simulink model "sf_tlbefore"  (Simulink 7.6)
settings: Solver=ode45  StartTime=0.0  StopTime=20  MaxStep=.01  RelTol=1e-3
settings Model: Creator=The MathWorks Inc.  CovMetricSettings=dcmtr  ExtModeAutoUpdateStatusClock=off
settings OptimizationCC: BooleanDataType=off  InlineInvariantSignals=on  InitFltsAndDblsToZero=on  EfficientMapNaN2IntZero=off
settings DebuggingCC: SaveWithParameterizedLinksMsg=none  SignalResolutionControl=TryResolveAllWithWarning  SolverPrmCheckMsg=none  MultiTaskDSMMsg=warning  MultiTaskCondExecSysMsg=none  StrictBusMsg=None
settings HardwareCC: TargetUnknown=on
settings SFSimCC: SimParseCustomCode=off
settings RTWCC: IncludeERTFirstTime=on
settings GRTTargetCC: TargetFcnLib=ansi_tfl_tmw.mat

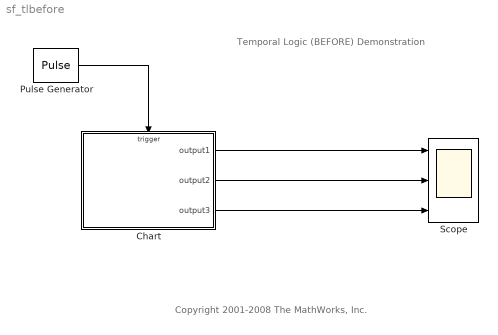
== system sf_tlbefore ==
  note: Temporal Logic (BEFORE) Demonstration
  note: Copyright 2001-2008 The MathWorks, Inc.
  Chart : Stateflow chart  TreatAsAtomicUnit=on
  Pulse Generator : DiscretePulseGenerator  PulseType=Time based  Period=1  PulseWidth=50
  Scope : Scope  NumInputPorts=3
      settings: TimeRange=20  YMin=0~0~-1  YMax=1.25~1.25~1
  wires:
  Pulse Generator/1 -> Chart/Trigger
  Chart/1(output1) -> Scope/1
  Chart/2(output2) -> Scope/2
  Chart/3(output3) -> Scope/3

== stateflow chart Chart ==
  state One [parallel]
    settings: executionOrder=1
    state A_state
      on count:signal_one++;
    A_state -> (junction 9) : before(10,count)[signal_one<5]{output1=1;}
    (junction 9) -> A_state
  state Two [parallel]
    settings: executionOrder=2
    state B_state
      on count:signal_two++;
    (junction 10) -> B_state
    B_state -> (junction 10) : before(20,count)[signal_two>10]{output2=1;}
  state Three [parallel]
    settings: executionOrder=3
    state C_state
      on count:signal_three++;
    C_state -> (junction 11) : before(10,count)[signal_three>11]{output3=1;}
    (junction 11) -> C_state
  (default) -> A_state : {signal_one=0;signal_two=0;signal_three=0;}
  data: output1 output double; signal_three local double; output2 output double; output3 output double; signal_one local double; signal_two local double
  events: count input RISING_EDGE_EVENT
